simulink model "svpwm"  (R2020b)
settings: Solver=VariableStepAuto  StartTime=0.0  StopTime=10.0  RelTol=1e-3
libraries: simulink x1
settings Model: Creator=Administrator  LastModifiedBy=Administrator
settings DataIOCC: ReturnWorkspaceOutputs=off
settings DebuggingCC: ArithmeticOperatorsInVariantConditions=warning
settings SFSimCC: SimUseLocalCustomCode=off  CustomCodeUndefinedFunction=UseInterfaceOnly
settings RTWCC: RTWUseLocalCustomCode=off
settings CodeAppCC: StateflowObjectComments=on
settings SimscapeCC: SimscapeNormalizeSystem=off

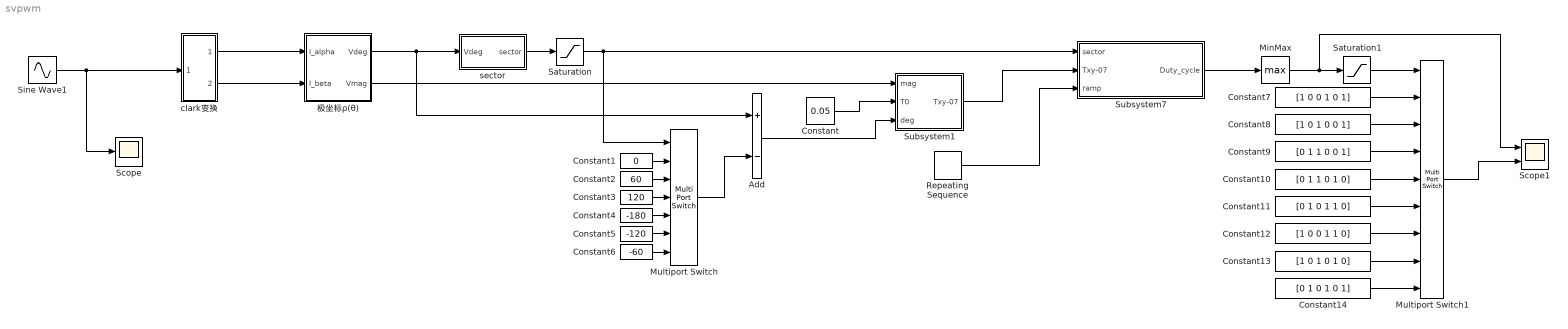
== system svpwm ==
  Add : Sum  Inputs=+-
  Constant : Constant  Value=0.05
  Constant1 : Constant  Value=0
  Constant10 : Constant  Value=[0 1 1 0 1 0]  VectorParams1D=off  SampleTime=-1
  Constant11 : Constant  Value=[0 1 0 1 1 0]  VectorParams1D=off  SampleTime=-1
  Constant12 : Constant  Value=[1 0 0 1 1 0]  VectorParams1D=off  SampleTime=-1
  Constant13 : Constant  Value=[1 0 1 0 1 0]  VectorParams1D=off  SampleTime=-1
  Constant14 : Constant  Value=[0 1 0 1 0 1]  VectorParams1D=off  SampleTime=-1
  Constant2 : Constant  Value=60
  Constant3 : Constant  Value=120
  Constant4 : Constant  Value=-180
  Constant5 : Constant  Value=-120
  Constant6 : Constant  Value=-60
  Constant7 : Constant  Value=[1 0 0 1 0 1]  VectorParams1D=off  SampleTime=-1
  Constant8 : Constant  Value=[1 0 1 0 0 1]  VectorParams1D=off  SampleTime=-1
  Constant9 : Constant  Value=[0 1 1 0 0 1]  VectorParams1D=off  SampleTime=-1
  MinMax : MinMax  Function=max
  Multiport Switch : MultiPortSwitch  Inputs=6
  Multiport Switch1 : MultiPortSwitch  Inputs=8
  Repeating Sequence : simulink/Sources/Repeating Sequence  rep_seq_t=[0 1e-4]  rep_seq_y=[0 1]
  Saturation : Saturate  UpperLimit=6  LowerLimit=1
  Saturation1 : Saturate  UpperLimit=8  LowerLimit=1
  Scope : Scope
  Scope1 : Scope  NumInputPorts=2
  Sine Wave1 : Sin  Amplitude=0.4  Frequency=2*pi*50  Phase=[0 -2*pi/3 2*pi/3]  SampleTime=1e-6
  Subsystem1 : Subsystem
  Subsystem7 : Subsystem
  clark变换 : Subsystem
  sector : Subsystem
  极坐标ρ(θ) : Subsystem
  wires:
  Sine Wave1/1 -> clark变换/1(I_abc), Scope/1
  clark变换/1(I_alpha) -> 极坐标ρ(θ)/1("I_alpha ")
  clark变换/2(I_beta) -> 极坐标ρ(θ)/2(I_beta)
  极坐标ρ(θ)/1(Vdeg) -> sector/1("Vdeg "), Add/1
  sector/1(sector) -> Saturation/1
  Saturation/1 -> Multiport Switch/1, Subsystem7/1(sector)
  Constant1/1 -> Multiport Switch/2
  Constant2/1 -> Multiport Switch/3
  Constant3/1 -> Multiport Switch/4
  Constant4/1 -> Multiport Switch/5
  Constant5/1 -> Multiport Switch/6
  Constant6/1 -> Multiport Switch/7
  Multiport Switch/1 -> Add/2
  极坐标ρ(θ)/2("Vmag ") -> Subsystem1/1(mag)
  Constant/1 -> Subsystem1/2("T0 ")
  Add/1 -> Subsystem1/3(deg)
  Subsystem1/1(Txy-07) -> Subsystem7/2(Txy-07)
  Repeating Sequence/1 -> Subsystem7/3(ramp)
  Subsystem7/1(Duty_cycle) -> MinMax/1
  MinMax/1 -> Scope1/1, Saturation1/1
  Saturation1/1 -> Multiport Switch1/1
  Constant7/1 -> Multiport Switch1/2
  Constant8/1 -> Multiport Switch1/3
  Constant14/1 -> Multiport Switch1/9
  Constant13/1 -> Multiport Switch1/8
  Constant12/1 -> Multiport Switch1/7
  Constant11/1 -> Multiport Switch1/6
  Constant10/1 -> Multiport Switch1/5
  Constant9/1 -> Multiport Switch1/4
  Multiport Switch1/1 -> Scope1/2

== system svpwm/Subsystem1 ==
  mag : Inport
  "T0 " : Inport  Port=2
  deg : Inport  Port=3
  Mux : Mux
  duty-cycles : Subsystem
  Txy-07 : Outport
  wires:
  duty-cycles/2(Ty) -> Mux/2
  duty-cycles/4(T7) -> Mux/4
  duty-cycles/1(Tx) -> Mux/1
  deg/1 -> duty-cycles/1(deg)
  "T0 "/1 -> duty-cycles/3("T0 ")
  Mux/1 -> Txy-07/1
  duty-cycles/3(T0) -> Mux/3
  mag/1 -> duty-cycles/2(mag)

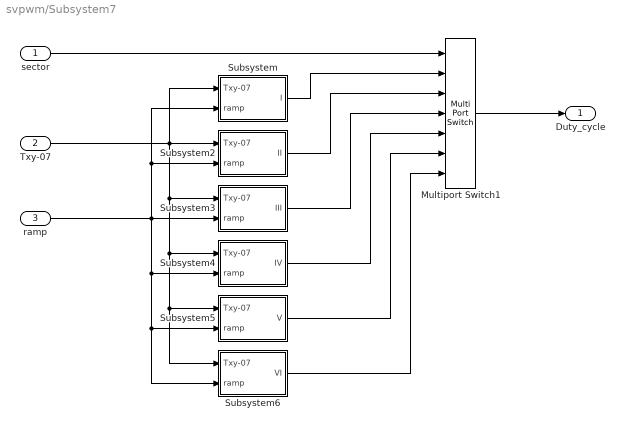
== system svpwm/Subsystem7 ==
  sector : Inport
  Txy-07 : Inport  Port=2
  ramp : Inport  Port=3
  Multiport Switch1 : MultiPortSwitch  Inputs=6
  Subsystem : Subsystem
  Subsystem2 : Subsystem
  Subsystem3 : Subsystem
  Subsystem4 : Subsystem
  Subsystem5 : Subsystem
  Subsystem6 : Subsystem
  Duty_cycle : Outport
  wires:
  Txy-07/1 -> Subsystem/1(Txy-07), Subsystem2/1(Txy-07), Subsystem3/1(Txy-07), Subsystem4/1(Txy-07), Subsystem5/1(Txy-07), Subsystem6/1(Txy-07)
  ramp/1 -> Subsystem/2(ramp), Subsystem2/2(ramp), Subsystem6/2(ramp), Subsystem5/2(ramp), Subsystem4/2(ramp), Subsystem3/2(ramp)
  Subsystem/1(I) -> Multiport Switch1/2
  Subsystem6/1(VI) -> Multiport Switch1/7
  Subsystem5/1(V) -> Multiport Switch1/6
  Subsystem3/1(III) -> Multiport Switch1/4
  Multiport Switch1/1 -> Duty_cycle/1
  Subsystem2/1(II) -> Multiport Switch1/3
  Subsystem4/1(IV) -> Multiport Switch1/5
  sector/1 -> Multiport Switch1/1

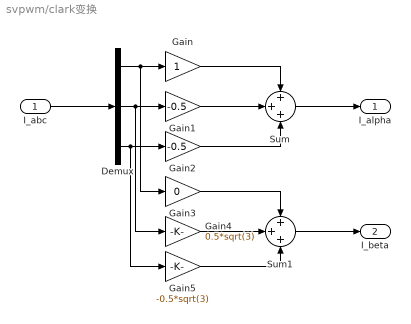
== system svpwm/clark变换 ==
  I_abc : Inport
  Demux : Demux  Outputs=3
  Gain : Gain
  Gain1 : Gain  Gain=-0.5
  Gain2 : Gain  Gain=-0.5
  Gain3 : Gain  Gain=0
  Gain4 : Gain  Gain=0.5*sqrt(3)
  Gain5 : Gain  Gain=-0.5*sqrt(3)
  Sum : Sum  Inputs=+++
  Sum1 : Sum  Inputs=+++
  I_alpha : Outport
  I_beta : Outport  Port=2
  wires:
  Gain5/1 -> Sum1/3
  Gain4/1 -> Sum1/2
  Gain1/1 -> Sum/2
  Gain2/1 -> Sum/3
  Demux/1 -> Gain/1, Gain3/1
  Sum/1 -> I_alpha/1
  I_abc/1 -> Demux/1
  Sum1/1 -> I_beta/1
  Demux/3 -> Gain5/1, Gain2/1
  Gain/1 -> Sum/1
  Demux/2 -> Gain4/1, Gain1/1
  Gain3/1 -> Sum1/1

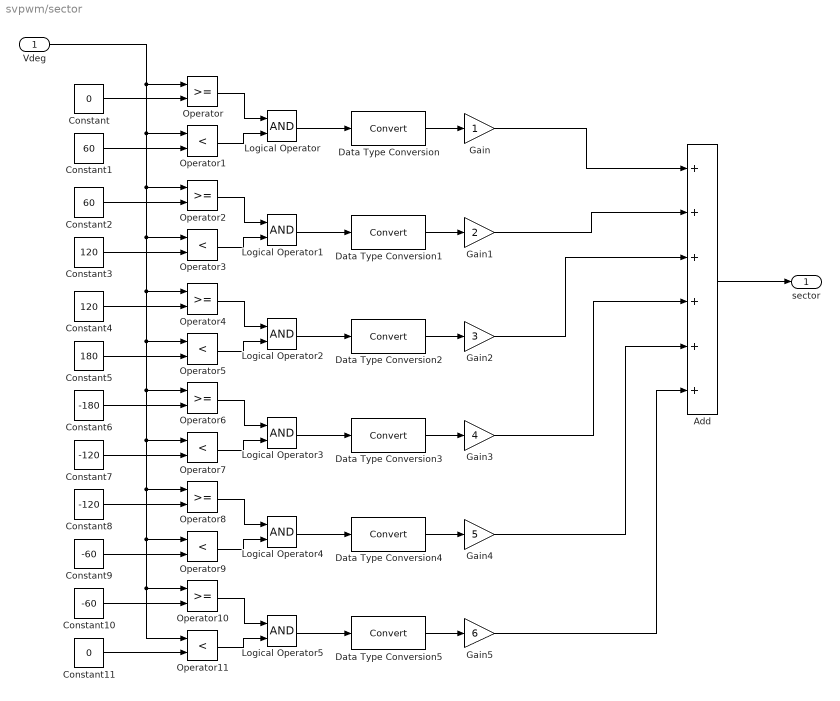
== system svpwm/sector ==
  "Vdeg " : Inport
  Add : Sum  Inputs=6
  Constant : Constant  Value=0
  Constant1 : Constant  Value=60
  Constant10 : Constant  Value=-60
  Constant11 : Constant  Value=0
  Constant2 : Constant  Value=60
  Constant3 : Constant  Value=120
  Constant4 : Constant  Value=120
  Constant5 : Constant  Value=180
  Constant6 : Constant  Value=-180
  Constant7 : Constant  Value=-120
  Constant8 : Constant  Value=-120
  Constant9 : Constant  Value=-60
  Data Type Conversion{,1..5} (6 alike) : DataTypeConversion
  Gain : Gain
  Gain1 : Gain  Gain=2
  Gain2 : Gain  Gain=3
  Gain3 : Gain  Gain=4
  Gain4 : Gain  Gain=5
  Gain5 : Gain  Gain=6
  Logical Operator{,1..5} (6 alike) : Logic  AllPortsSameDT=off  OutDataTypeStr=boolean
  Operator{,2,4,6,8,10} (6 alike) : RelationalOperator  OutDataTypeStr=boolean  RndMeth=Simplest
  Operator{1,3,5,7,9,11} (6 alike) : RelationalOperator  Operator=<  OutDataTypeStr=boolean  RndMeth=Simplest
  sector : Outport
  wires:
  Gain3/1 -> Add/4
  Gain1/1 -> Add/2
  Operator10/1 -> Logical Operator5/1
  Operator11/1 -> Logical Operator5/2
  "Vdeg "/1 -> Operator2/1, Operator6/1, Operator10/1, Operator11/1, Operator9/1, Operator8/1, Operator7/1, Operator5/1, Operator4/1, Operator3/1, Operator1/1, Operator/1
  Constant10/1 -> Operator10/2
  Logical Operator5/1 -> Data Type Conversion5/1
  Data Type Conversion5/1 -> Gain5/1
  Constant2/1 -> Operator2/2
  Operator2/1 -> Logical Operator1/1
  Constant3/1 -> Operator3/2
  Logical Operator1/1 -> Data Type Conversion1/1
  Operator3/1 -> Logical Operator1/2
  Data Type Conversion1/1 -> Gain1/1
  Logical Operator/1 -> Data Type Conversion/1
  Constant11/1 -> Operator11/2
  Constant/1 -> Operator/2
  Operator/1 -> Logical Operator/1
  Constant1/1 -> Operator1/2
  Gain/1 -> Add/1
  Operator1/1 -> Logical Operator/2
  Operator4/1 -> Logical Operator2/1
  Logical Operator2/1 -> Data Type Conversion2/1
  Constant5/1 -> Operator5/2
  Constant4/1 -> Operator4/2
  Operator5/1 -> Logical Operator2/2
  Data Type Conversion2/1 -> Gain2/1
  Constant7/1 -> Operator7/2
  Operator6/1 -> Logical Operator3/1
  Data Type Conversion3/1 -> Gain3/1
  Constant6/1 -> Operator6/2
  Operator7/1 -> Logical Operator3/2
  Logical Operator3/1 -> Data Type Conversion3/1
  Gain4/1 -> Add/5
  Gain5/1 -> Add/6
  Gain2/1 -> Add/3
  Data Type Conversion/1 -> Gain/1
  Add/1 -> sector/1
  Constant9/1 -> Operator9/2
  Operator8/1 -> Logical Operator4/1
  Operator9/1 -> Logical Operator4/2
  Data Type Conversion4/1 -> Gain4/1
  Logical Operator4/1 -> Data Type Conversion4/1
  Constant8/1 -> Operator8/2

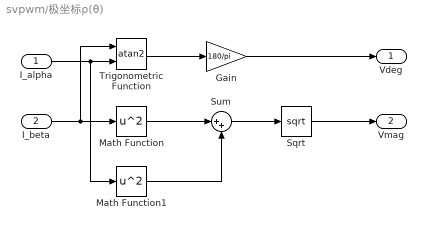
== system svpwm/极坐标ρ(θ) ==
  "I_alpha " : Inport
  I_beta : Inport  Port=2
  Gain : Gain  Gain=180/pi
  Math Function : Math  Operator=square  SignedPower=on  SaturateOnIntegerOverflow=on
  Math Function1 : Math  Operator=square  SignedPower=on  SaturateOnIntegerOverflow=on
  Sqrt : Sqrt  SaturateOnIntegerOverflow=on
  Sum : Sum  Inputs=|++
  Trigonometric Function : Trigonometry  Operator=atan2
  Vdeg : Outport
  "Vmag " : Outport  Port=2
  wires:
  "I_alpha "/1 -> Math Function1/1, Trigonometric Function/2
  I_beta/1 -> Trigonometric Function/1, Math Function/1
  Math Function/1 -> Sum/1
  Math Function1/1 -> Sum/2
  Sum/1 -> Sqrt/1
  Gain/1 -> Vdeg/1
  Trigonometric Function/1 -> Gain/1
  Sqrt/1 -> "Vmag "/1

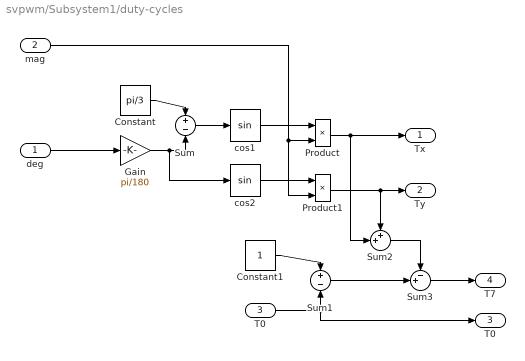
== system svpwm/Subsystem1/duty-cycles ==
  deg : Inport
  mag : Inport  Port=2
  "T0 " : Inport  Port=3
  Constant : Constant  Value=pi/3
  Constant1 : Constant
  Gain : Gain  Gain=pi/180
  Product : Product
  Product1 : Product
  Sum : Sum  Inputs=+|-
  Sum1 : Sum  Inputs=+-
  Sum2 : Sum  Inputs=++|
  Sum3 : Sum  Inputs=-+|
  cos1 : Trigonometry
  cos2 : Trigonometry
  Tx : Outport
  Ty : Outport  Port=2
  T0 : Outport  Port=3
  T7 : Outport  Port=4
  wires:
  Gain/1 -> cos2/1, Sum/2
  cos1/1 -> Product/1
  Sum/1 -> cos1/1
  mag/1 -> Product1/2, Product/2
  deg/1 -> Gain/1
  Product1/1 -> Sum2/1, Ty/1
  Product/1 -> Sum2/2, Tx/1
  cos2/1 -> Product1/1
  Constant/1 -> Sum/1
  Constant1/1 -> Sum1/1
  "T0 "/1 -> Sum1/2, T0/1
  Sum1/1 -> Sum3/2
  Sum2/1 -> Sum3/1
  Sum3/1 -> T7/1

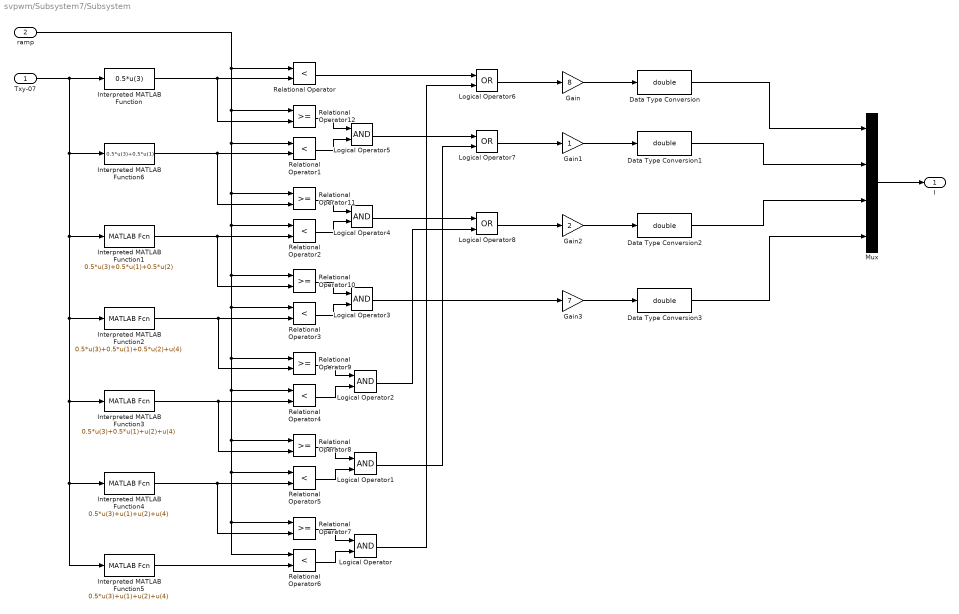
== system svpwm/Subsystem7/Subsystem ==
  Txy-07 : Inport
  ramp : Inport  Port=2
  Data Type Conversion{,1..3} (4 alike) : DataTypeConversion  OutDataTypeStr=double
  Gain : Gain  Gain=8
  Gain1 : Gain
  Gain2 : Gain  Gain=2
  Gain3 : Gain  Gain=7
  Interpreted MATLAB Function : MATLABFcn  MATLABFcn=0.5*u(3)
  Interpreted MATLAB Function1 : MATLABFcn  MATLABFcn=0.5*u(3)+0.5*u(1)+0.5*u(2)
  Interpreted MATLAB Function2 : MATLABFcn  MATLABFcn=0.5*u(3)+0.5*u(1)+0.5*u(2)+u(4)
  Interpreted MATLAB Function3 : MATLABFcn  MATLABFcn=0.5*u(3)+0.5*u(1)+u(2)+u(4)
  Interpreted MATLAB Function4 : MATLABFcn  MATLABFcn=0.5*u(3)+u(1)+u(2)+u(4)
  Interpreted MATLAB Function5 : MATLABFcn  MATLABFcn=0.5*u(3)+u(1)+u(2)+u(4)
  Interpreted MATLAB Function6 : MATLABFcn  MATLABFcn=0.5*u(3)+0.5*u(1)
  Logical Operator{,1..5} (6 alike) : Logic  AllPortsSameDT=off  OutDataTypeStr=boolean
  Logical Operator6 : Logic  Operator=OR  AllPortsSameDT=off  OutDataTypeStr=boolean
  Logical Operator7 : Logic  Operator=OR  AllPortsSameDT=off  OutDataTypeStr=boolean
  Logical Operator8 : Logic  Operator=OR  AllPortsSameDT=off  OutDataTypeStr=boolean
  Mux : Mux
  Relational Operator{,1..6} (7 alike) : RelationalOperator  Operator=<  OutDataTypeStr=boolean  RndMeth=Simplest
  Relational Operator{7..12} (6 alike) : RelationalOperator  OutDataTypeStr=boolean  RndMeth=Simplest
  I : Outport
  wires:
  Txy-07/1 -> Interpreted MATLAB Function5/1, Interpreted MATLAB Function4/1, Interpreted MATLAB Function3/1, Interpreted MATLAB Function2/1, Interpreted MATLAB Function1/1, Interpreted MATLAB Function6/1, Interpreted MATLAB Function/1
  Interpreted MATLAB Function/1 -> Relational Operator12/2, Relational Operator/2
  Interpreted MATLAB Function6/1 -> Relational Operator11/2, Relational Operator1/2
  Interpreted MATLAB Function1/1 -> Relational Operator10/2, Relational Operator2/2
  Interpreted MATLAB Function2/1 -> Relational Operator9/2, Relational Operator3/2
  Interpreted MATLAB Function3/1 -> Relational Operator8/2, Relational Operator4/2
  Interpreted MATLAB Function5/1 -> Relational Operator6/2
  Interpreted MATLAB Function4/1 -> Relational Operator7/2, Relational Operator5/2
  Relational Operator7/1 -> Logical Operator/1
  Relational Operator6/1 -> Logical Operator/2
  Relational Operator12/1 -> Logical Operator5/1
  Relational Operator1/1 -> Logical Operator5/2
  Relational Operator11/1 -> Logical Operator4/1
  Relational Operator2/1 -> Logical Operator4/2
  Relational Operator10/1 -> Logical Operator3/1
  Relational Operator3/1 -> Logical Operator3/2
  Relational Operator9/1 -> Logical Operator2/1
  Relational Operator4/1 -> Logical Operator2/2
  Relational Operator8/1 -> Logical Operator1/1
  Relational Operator5/1 -> Logical Operator1/2
  ramp/1 -> Relational Operator12/1, Relational Operator11/1, Relational Operator10/1, Relational Operator9/1, Relational Operator8/1, Relational Operator7/1, Relational Operator6/1, Relational Operator5/1, Relational Operator4/1, Relational Operator3/1, Relational Operator2/1, Relational Operator1/1, Relational Operator/1
  Relational Operator/1 -> Logical Operator6/1
  Logical Operator/1 -> Logical Operator6/2
  Logical Operator5/1 -> Logical Operator7/1
  Logical Operator1/1 -> Logical Operator7/2
  Logical Operator4/1 -> Logical Operator8/1
  Logical Operator2/1 -> Logical Operator8/2
  Logical Operator6/1 -> Gain/1
  Logical Operator7/1 -> Gain1/1
  Logical Operator8/1 -> Gain2/1
  Logical Operator3/1 -> Gain3/1
  Gain3/1 -> Data Type Conversion3/1
  Gain2/1 -> Data Type Conversion2/1
  Gain1/1 -> Data Type Conversion1/1
  Gain/1 -> Data Type Conversion/1
  Data Type Conversion/1 -> Mux/1
  Data Type Conversion1/1 -> Mux/2
  Data Type Conversion2/1 -> Mux/3
  Data Type Conversion3/1 -> Mux/4
  Mux/1 -> I/1

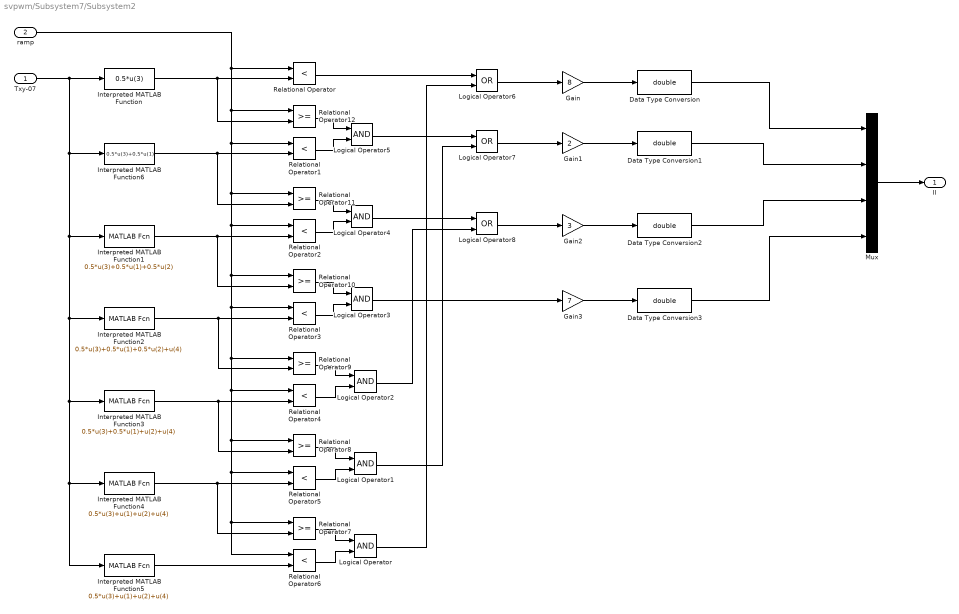
== system svpwm/Subsystem7/Subsystem2 ==
  Txy-07 : Inport
  ramp : Inport  Port=2
  Data Type Conversion{,1..3} (4 alike) : DataTypeConversion  OutDataTypeStr=double
  Gain : Gain  Gain=8
  Gain1 : Gain  Gain=2
  Gain2 : Gain  Gain=3
  Gain3 : Gain  Gain=7
  Interpreted MATLAB Function : MATLABFcn  MATLABFcn=0.5*u(3)
  Interpreted MATLAB Function1 : MATLABFcn  MATLABFcn=0.5*u(3)+0.5*u(1)+0.5*u(2)
  Interpreted MATLAB Function2 : MATLABFcn  MATLABFcn=0.5*u(3)+0.5*u(1)+0.5*u(2)+u(4)
  Interpreted MATLAB Function3 : MATLABFcn  MATLABFcn=0.5*u(3)+0.5*u(1)+u(2)+u(4)
  Interpreted MATLAB Function4 : MATLABFcn  MATLABFcn=0.5*u(3)+u(1)+u(2)+u(4)
  Interpreted MATLAB Function5 : MATLABFcn  MATLABFcn=0.5*u(3)+u(1)+u(2)+u(4)
  Interpreted MATLAB Function6 : MATLABFcn  MATLABFcn=0.5*u(3)+0.5*u(1)
  Logical Operator{,1..5} (6 alike) : Logic  AllPortsSameDT=off  OutDataTypeStr=boolean
  Logical Operator6 : Logic  Operator=OR  AllPortsSameDT=off  OutDataTypeStr=boolean
  Logical Operator7 : Logic  Operator=OR  AllPortsSameDT=off  OutDataTypeStr=boolean
  Logical Operator8 : Logic  Operator=OR  AllPortsSameDT=off  OutDataTypeStr=boolean
  Mux : Mux
  Relational Operator{,1..6} (7 alike) : RelationalOperator  Operator=<  OutDataTypeStr=boolean  RndMeth=Simplest
  Relational Operator{7..12} (6 alike) : RelationalOperator  OutDataTypeStr=boolean  RndMeth=Simplest
  II : Outport
  wires:
  Mux/1 -> II/1
  Data Type Conversion3/1 -> Mux/4
  Data Type Conversion2/1 -> Mux/3
  Data Type Conversion1/1 -> Mux/2
  Data Type Conversion/1 -> Mux/1
  Gain/1 -> Data Type Conversion/1
  Gain1/1 -> Data Type Conversion1/1
  Gain2/1 -> Data Type Conversion2/1
  Gain3/1 -> Data Type Conversion3/1
  Logical Operator3/1 -> Gain3/1
  Logical Operator8/1 -> Gain2/1
  Logical Operator7/1 -> Gain1/1
  Logical Operator6/1 -> Gain/1
  Logical Operator2/1 -> Logical Operator8/2
  Logical Operator4/1 -> Logical Operator8/1
  Logical Operator1/1 -> Logical Operator7/2
  Logical Operator5/1 -> Logical Operator7/1
  Logical Operator/1 -> Logical Operator6/2
  Relational Operator/1 -> Logical Operator6/1
  ramp/1 -> Relational Operator/1, Relational Operator1/1, Relational Operator2/1, Relational Operator3/1, Relational Operator4/1, Relational Operator5/1, Relational Operator6/1, Relational Operator7/1, Relational Operator8/1, Relational Operator9/1, Relational Operator10/1, Relational Operator11/1, Relational Operator12/1
  Relational Operator5/1 -> Logical Operator1/2
  Relational Operator8/1 -> Logical Operator1/1
  Relational Operator4/1 -> Logical Operator2/2
  Relational Operator9/1 -> Logical Operator2/1
  Relational Operator3/1 -> Logical Operator3/2
  Relational Operator10/1 -> Logical Operator3/1
  Relational Operator2/1 -> Logical Operator4/2
  Relational Operator11/1 -> Logical Operator4/1
  Relational Operator1/1 -> Logical Operator5/2
  Relational Operator12/1 -> Logical Operator5/1
  Relational Operator6/1 -> Logical Operator/2
  Relational Operator7/1 -> Logical Operator/1
  Interpreted MATLAB Function4/1 -> Relational Operator5/2, Relational Operator7/2
  Interpreted MATLAB Function5/1 -> Relational Operator6/2
  Interpreted MATLAB Function3/1 -> Relational Operator4/2, Relational Operator8/2
  Interpreted MATLAB Function2/1 -> Relational Operator3/2, Relational Operator9/2
  Interpreted MATLAB Function1/1 -> Relational Operator2/2, Relational Operator10/2
  Interpreted MATLAB Function6/1 -> Relational Operator1/2, Relational Operator11/2
  Interpreted MATLAB Function/1 -> Relational Operator/2, Relational Operator12/2
  Txy-07/1 -> Interpreted MATLAB Function/1, Interpreted MATLAB Function6/1, Interpreted MATLAB Function1/1, Interpreted MATLAB Function2/1, Interpreted MATLAB Function3/1, Interpreted MATLAB Function4/1, Interpreted MATLAB Function5/1

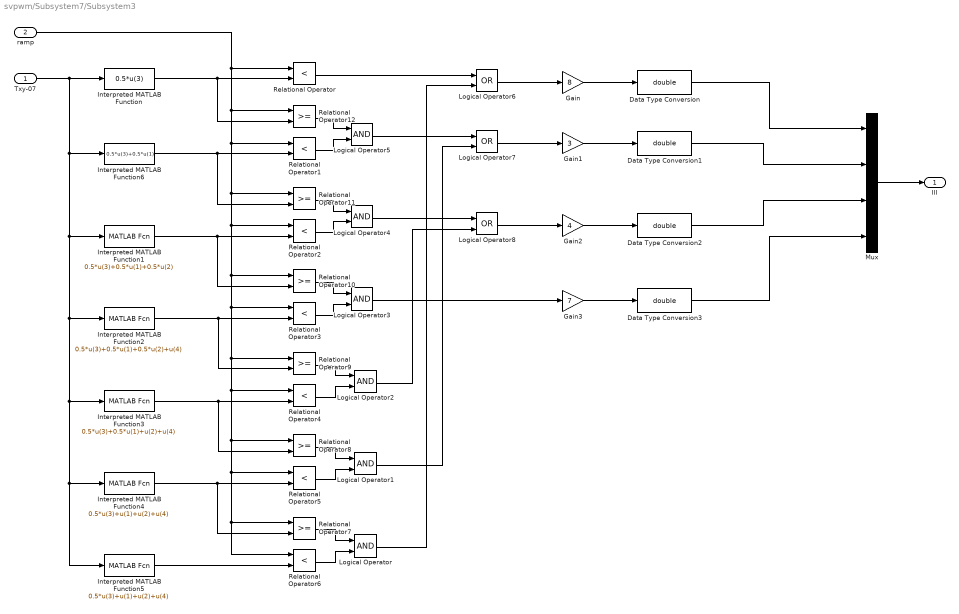
== system svpwm/Subsystem7/Subsystem3 ==
  Txy-07 : Inport
  ramp : Inport  Port=2
  Data Type Conversion{,1..3} (4 alike) : DataTypeConversion  OutDataTypeStr=double
  Gain : Gain  Gain=8
  Gain1 : Gain  Gain=3
  Gain2 : Gain  Gain=4
  Gain3 : Gain  Gain=7
  Interpreted MATLAB Function : MATLABFcn  MATLABFcn=0.5*u(3)
  Interpreted MATLAB Function1 : MATLABFcn  MATLABFcn=0.5*u(3)+0.5*u(1)+0.5*u(2)
  Interpreted MATLAB Function2 : MATLABFcn  MATLABFcn=0.5*u(3)+0.5*u(1)+0.5*u(2)+u(4)
  Interpreted MATLAB Function3 : MATLABFcn  MATLABFcn=0.5*u(3)+0.5*u(1)+u(2)+u(4)
  Interpreted MATLAB Function4 : MATLABFcn  MATLABFcn=0.5*u(3)+u(1)+u(2)+u(4)
  Interpreted MATLAB Function5 : MATLABFcn  MATLABFcn=0.5*u(3)+u(1)+u(2)+u(4)
  Interpreted MATLAB Function6 : MATLABFcn  MATLABFcn=0.5*u(3)+0.5*u(1)
  Logical Operator{,1..5} (6 alike) : Logic  AllPortsSameDT=off  OutDataTypeStr=boolean
  Logical Operator6 : Logic  Operator=OR  AllPortsSameDT=off  OutDataTypeStr=boolean
  Logical Operator7 : Logic  Operator=OR  AllPortsSameDT=off  OutDataTypeStr=boolean
  Logical Operator8 : Logic  Operator=OR  AllPortsSameDT=off  OutDataTypeStr=boolean
  Mux : Mux
  Relational Operator{,1..6} (7 alike) : RelationalOperator  Operator=<  OutDataTypeStr=boolean  RndMeth=Simplest
  Relational Operator{7..12} (6 alike) : RelationalOperator  OutDataTypeStr=boolean  RndMeth=Simplest
  III : Outport
  wires:
  Txy-07/1 -> Interpreted MATLAB Function5/1, Interpreted MATLAB Function4/1, Interpreted MATLAB Function3/1, Interpreted MATLAB Function2/1, Interpreted MATLAB Function1/1, Interpreted MATLAB Function6/1, Interpreted MATLAB Function/1
  Interpreted MATLAB Function/1 -> Relational Operator12/2, Relational Operator/2
  Interpreted MATLAB Function6/1 -> Relational Operator11/2, Relational Operator1/2
  Interpreted MATLAB Function1/1 -> Relational Operator10/2, Relational Operator2/2
  Interpreted MATLAB Function2/1 -> Relational Operator9/2, Relational Operator3/2
  Interpreted MATLAB Function3/1 -> Relational Operator8/2, Relational Operator4/2
  Interpreted MATLAB Function5/1 -> Relational Operator6/2
  Interpreted MATLAB Function4/1 -> Relational Operator7/2, Relational Operator5/2
  Relational Operator7/1 -> Logical Operator/1
  Relational Operator6/1 -> Logical Operator/2
  Relational Operator12/1 -> Logical Operator5/1
  Relational Operator1/1 -> Logical Operator5/2
  Relational Operator11/1 -> Logical Operator4/1
  Relational Operator2/1 -> Logical Operator4/2
  Relational Operator10/1 -> Logical Operator3/1
  Relational Operator3/1 -> Logical Operator3/2
  Relational Operator9/1 -> Logical Operator2/1
  Relational Operator4/1 -> Logical Operator2/2
  Relational Operator8/1 -> Logical Operator1/1
  Relational Operator5/1 -> Logical Operator1/2
  ramp/1 -> Relational Operator12/1, Relational Operator11/1, Relational Operator10/1, Relational Operator9/1, Relational Operator8/1, Relational Operator7/1, Relational Operator6/1, Relational Operator5/1, Relational Operator4/1, Relational Operator3/1, Relational Operator2/1, Relational Operator1/1, Relational Operator/1
  Relational Operator/1 -> Logical Operator6/1
  Logical Operator/1 -> Logical Operator6/2
  Logical Operator5/1 -> Logical Operator7/1
  Logical Operator1/1 -> Logical Operator7/2
  Logical Operator4/1 -> Logical Operator8/1
  Logical Operator2/1 -> Logical Operator8/2
  Logical Operator6/1 -> Gain/1
  Logical Operator7/1 -> Gain1/1
  Logical Operator8/1 -> Gain2/1
  Logical Operator3/1 -> Gain3/1
  Gain3/1 -> Data Type Conversion3/1
  Gain2/1 -> Data Type Conversion2/1
  Gain1/1 -> Data Type Conversion1/1
  Gain/1 -> Data Type Conversion/1
  Data Type Conversion/1 -> Mux/1
  Data Type Conversion1/1 -> Mux/2
  Data Type Conversion2/1 -> Mux/3
  Data Type Conversion3/1 -> Mux/4
  Mux/1 -> III/1

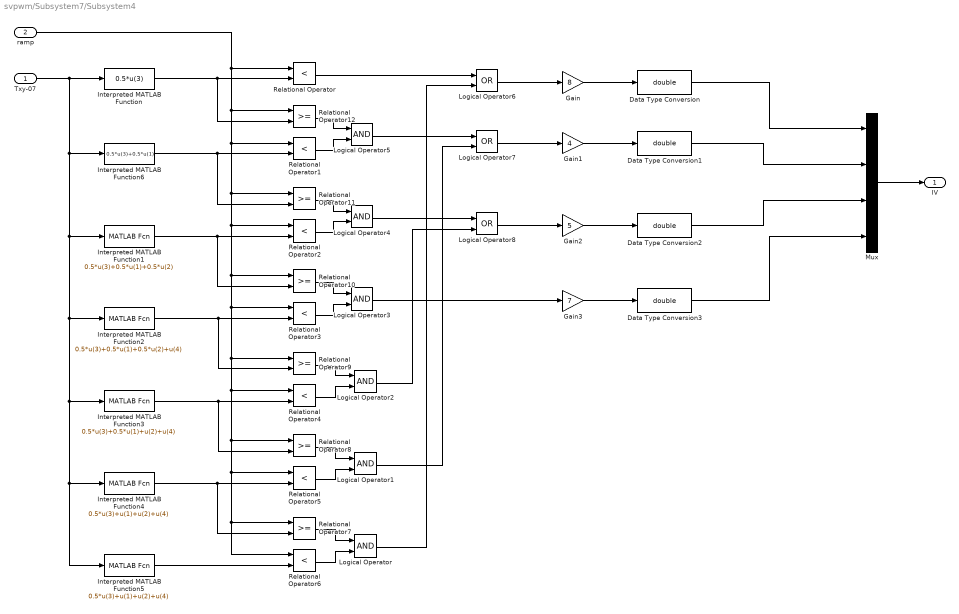
== system svpwm/Subsystem7/Subsystem4 ==
  Txy-07 : Inport
  ramp : Inport  Port=2
  Data Type Conversion{,1..3} (4 alike) : DataTypeConversion  OutDataTypeStr=double
  Gain : Gain  Gain=8
  Gain1 : Gain  Gain=4
  Gain2 : Gain  Gain=5
  Gain3 : Gain  Gain=7
  Interpreted MATLAB Function : MATLABFcn  MATLABFcn=0.5*u(3)
  Interpreted MATLAB Function1 : MATLABFcn  MATLABFcn=0.5*u(3)+0.5*u(1)+0.5*u(2)
  Interpreted MATLAB Function2 : MATLABFcn  MATLABFcn=0.5*u(3)+0.5*u(1)+0.5*u(2)+u(4)
  Interpreted MATLAB Function3 : MATLABFcn  MATLABFcn=0.5*u(3)+0.5*u(1)+u(2)+u(4)
  Interpreted MATLAB Function4 : MATLABFcn  MATLABFcn=0.5*u(3)+u(1)+u(2)+u(4)
  Interpreted MATLAB Function5 : MATLABFcn  MATLABFcn=0.5*u(3)+u(1)+u(2)+u(4)
  Interpreted MATLAB Function6 : MATLABFcn  MATLABFcn=0.5*u(3)+0.5*u(1)
  Logical Operator{,1..5} (6 alike) : Logic  AllPortsSameDT=off  OutDataTypeStr=boolean
  Logical Operator6 : Logic  Operator=OR  AllPortsSameDT=off  OutDataTypeStr=boolean
  Logical Operator7 : Logic  Operator=OR  AllPortsSameDT=off  OutDataTypeStr=boolean
  Logical Operator8 : Logic  Operator=OR  AllPortsSameDT=off  OutDataTypeStr=boolean
  Mux : Mux
  Relational Operator{,1..6} (7 alike) : RelationalOperator  Operator=<  OutDataTypeStr=boolean  RndMeth=Simplest
  Relational Operator{7..12} (6 alike) : RelationalOperator  OutDataTypeStr=boolean  RndMeth=Simplest
  IV : Outport
  wires:
  Mux/1 -> IV/1
  Data Type Conversion3/1 -> Mux/4
  Data Type Conversion2/1 -> Mux/3
  Data Type Conversion1/1 -> Mux/2
  Data Type Conversion/1 -> Mux/1
  Gain/1 -> Data Type Conversion/1
  Gain1/1 -> Data Type Conversion1/1
  Gain2/1 -> Data Type Conversion2/1
  Gain3/1 -> Data Type Conversion3/1
  Logical Operator3/1 -> Gain3/1
  Logical Operator8/1 -> Gain2/1
  Logical Operator7/1 -> Gain1/1
  Logical Operator6/1 -> Gain/1
  Logical Operator2/1 -> Logical Operator8/2
  Logical Operator4/1 -> Logical Operator8/1
  Logical Operator1/1 -> Logical Operator7/2
  Logical Operator5/1 -> Logical Operator7/1
  Logical Operator/1 -> Logical Operator6/2
  Relational Operator/1 -> Logical Operator6/1
  ramp/1 -> Relational Operator/1, Relational Operator1/1, Relational Operator2/1, Relational Operator3/1, Relational Operator4/1, Relational Operator5/1, Relational Operator6/1, Relational Operator7/1, Relational Operator8/1, Relational Operator9/1, Relational Operator10/1, Relational Operator11/1, Relational Operator12/1
  Relational Operator5/1 -> Logical Operator1/2
  Relational Operator8/1 -> Logical Operator1/1
  Relational Operator4/1 -> Logical Operator2/2
  Relational Operator9/1 -> Logical Operator2/1
  Relational Operator3/1 -> Logical Operator3/2
  Relational Operator10/1 -> Logical Operator3/1
  Relational Operator2/1 -> Logical Operator4/2
  Relational Operator11/1 -> Logical Operator4/1
  Relational Operator1/1 -> Logical Operator5/2
  Relational Operator12/1 -> Logical Operator5/1
  Relational Operator6/1 -> Logical Operator/2
  Relational Operator7/1 -> Logical Operator/1
  Interpreted MATLAB Function4/1 -> Relational Operator5/2, Relational Operator7/2
  Interpreted MATLAB Function5/1 -> Relational Operator6/2
  Interpreted MATLAB Function3/1 -> Relational Operator4/2, Relational Operator8/2
  Interpreted MATLAB Function2/1 -> Relational Operator3/2, Relational Operator9/2
  Interpreted MATLAB Function1/1 -> Relational Operator2/2, Relational Operator10/2
  Interpreted MATLAB Function6/1 -> Relational Operator1/2, Relational Operator11/2
  Interpreted MATLAB Function/1 -> Relational Operator/2, Relational Operator12/2
  Txy-07/1 -> Interpreted MATLAB Function/1, Interpreted MATLAB Function6/1, Interpreted MATLAB Function1/1, Interpreted MATLAB Function2/1, Interpreted MATLAB Function3/1, Interpreted MATLAB Function4/1, Interpreted MATLAB Function5/1

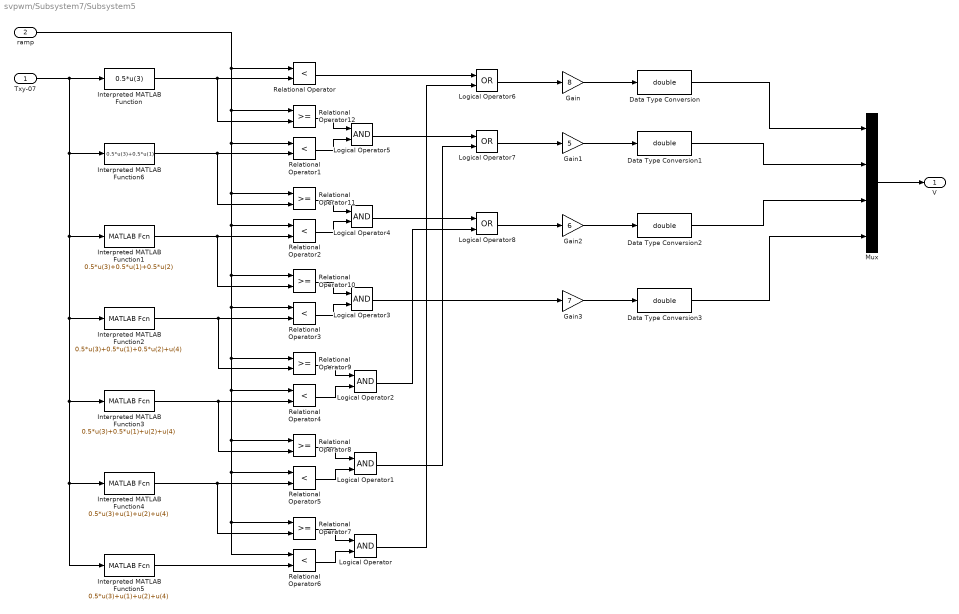
== system svpwm/Subsystem7/Subsystem5 ==
  Txy-07 : Inport
  ramp : Inport  Port=2
  Data Type Conversion{,1..3} (4 alike) : DataTypeConversion  OutDataTypeStr=double
  Gain : Gain  Gain=8
  Gain1 : Gain  Gain=5
  Gain2 : Gain  Gain=6
  Gain3 : Gain  Gain=7
  Interpreted MATLAB Function : MATLABFcn  MATLABFcn=0.5*u(3)
  Interpreted MATLAB Function1 : MATLABFcn  MATLABFcn=0.5*u(3)+0.5*u(1)+0.5*u(2)
  Interpreted MATLAB Function2 : MATLABFcn  MATLABFcn=0.5*u(3)+0.5*u(1)+0.5*u(2)+u(4)
  Interpreted MATLAB Function3 : MATLABFcn  MATLABFcn=0.5*u(3)+0.5*u(1)+u(2)+u(4)
  Interpreted MATLAB Function4 : MATLABFcn  MATLABFcn=0.5*u(3)+u(1)+u(2)+u(4)
  Interpreted MATLAB Function5 : MATLABFcn  MATLABFcn=0.5*u(3)+u(1)+u(2)+u(4)
  Interpreted MATLAB Function6 : MATLABFcn  MATLABFcn=0.5*u(3)+0.5*u(1)
  Logical Operator{,1..5} (6 alike) : Logic  AllPortsSameDT=off  OutDataTypeStr=boolean
  Logical Operator6 : Logic  Operator=OR  AllPortsSameDT=off  OutDataTypeStr=boolean
  Logical Operator7 : Logic  Operator=OR  AllPortsSameDT=off  OutDataTypeStr=boolean
  Logical Operator8 : Logic  Operator=OR  AllPortsSameDT=off  OutDataTypeStr=boolean
  Mux : Mux
  Relational Operator{,1..6} (7 alike) : RelationalOperator  Operator=<  OutDataTypeStr=boolean  RndMeth=Simplest
  Relational Operator{7..12} (6 alike) : RelationalOperator  OutDataTypeStr=boolean  RndMeth=Simplest
  V : Outport
  wires:
  Txy-07/1 -> Interpreted MATLAB Function5/1, Interpreted MATLAB Function4/1, Interpreted MATLAB Function3/1, Interpreted MATLAB Function2/1, Interpreted MATLAB Function1/1, Interpreted MATLAB Function6/1, Interpreted MATLAB Function/1
  Interpreted MATLAB Function/1 -> Relational Operator12/2, Relational Operator/2
  Interpreted MATLAB Function6/1 -> Relational Operator11/2, Relational Operator1/2
  Interpreted MATLAB Function1/1 -> Relational Operator10/2, Relational Operator2/2
  Interpreted MATLAB Function2/1 -> Relational Operator9/2, Relational Operator3/2
  Interpreted MATLAB Function3/1 -> Relational Operator8/2, Relational Operator4/2
  Interpreted MATLAB Function5/1 -> Relational Operator6/2
  Interpreted MATLAB Function4/1 -> Relational Operator7/2, Relational Operator5/2
  Relational Operator7/1 -> Logical Operator/1
  Relational Operator6/1 -> Logical Operator/2
  Relational Operator12/1 -> Logical Operator5/1
  Relational Operator1/1 -> Logical Operator5/2
  Relational Operator11/1 -> Logical Operator4/1
  Relational Operator2/1 -> Logical Operator4/2
  Relational Operator10/1 -> Logical Operator3/1
  Relational Operator3/1 -> Logical Operator3/2
  Relational Operator9/1 -> Logical Operator2/1
  Relational Operator4/1 -> Logical Operator2/2
  Relational Operator8/1 -> Logical Operator1/1
  Relational Operator5/1 -> Logical Operator1/2
  ramp/1 -> Relational Operator12/1, Relational Operator11/1, Relational Operator10/1, Relational Operator9/1, Relational Operator8/1, Relational Operator7/1, Relational Operator6/1, Relational Operator5/1, Relational Operator4/1, Relational Operator3/1, Relational Operator2/1, Relational Operator1/1, Relational Operator/1
  Relational Operator/1 -> Logical Operator6/1
  Logical Operator/1 -> Logical Operator6/2
  Logical Operator5/1 -> Logical Operator7/1
  Logical Operator1/1 -> Logical Operator7/2
  Logical Operator4/1 -> Logical Operator8/1
  Logical Operator2/1 -> Logical Operator8/2
  Logical Operator6/1 -> Gain/1
  Logical Operator7/1 -> Gain1/1
  Logical Operator8/1 -> Gain2/1
  Logical Operator3/1 -> Gain3/1
  Gain3/1 -> Data Type Conversion3/1
  Gain2/1 -> Data Type Conversion2/1
  Gain1/1 -> Data Type Conversion1/1
  Gain/1 -> Data Type Conversion/1
  Data Type Conversion/1 -> Mux/1
  Data Type Conversion1/1 -> Mux/2
  Data Type Conversion2/1 -> Mux/3
  Data Type Conversion3/1 -> Mux/4
  Mux/1 -> V/1

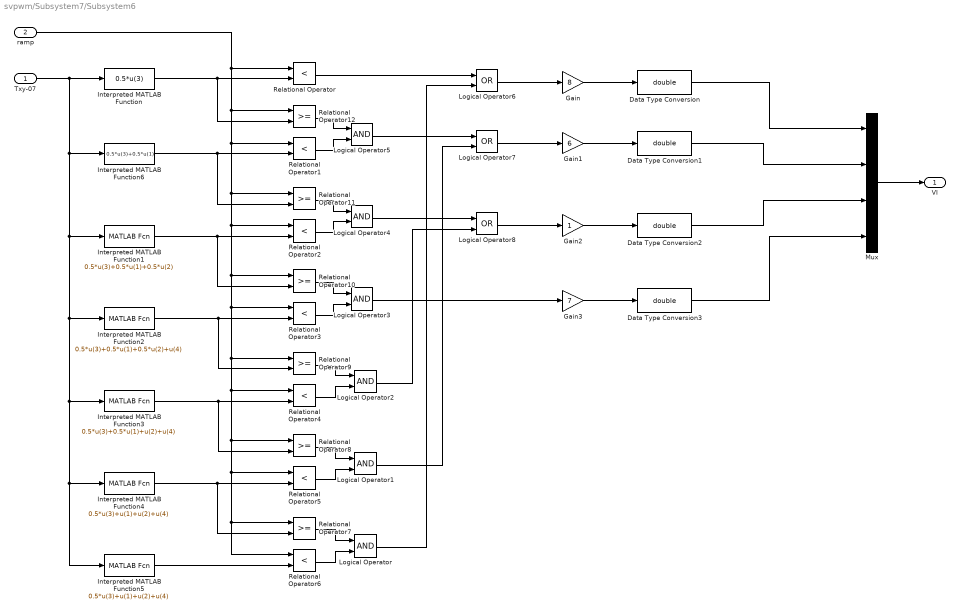
== system svpwm/Subsystem7/Subsystem6 ==
  Txy-07 : Inport
  ramp : Inport  Port=2
  Data Type Conversion{,1..3} (4 alike) : DataTypeConversion  OutDataTypeStr=double
  Gain : Gain  Gain=8
  Gain1 : Gain  Gain=6
  Gain2 : Gain
  Gain3 : Gain  Gain=7
  Interpreted MATLAB Function : MATLABFcn  MATLABFcn=0.5*u(3)
  Interpreted MATLAB Function1 : MATLABFcn  MATLABFcn=0.5*u(3)+0.5*u(1)+0.5*u(2)
  Interpreted MATLAB Function2 : MATLABFcn  MATLABFcn=0.5*u(3)+0.5*u(1)+0.5*u(2)+u(4)
  Interpreted MATLAB Function3 : MATLABFcn  MATLABFcn=0.5*u(3)+0.5*u(1)+u(2)+u(4)
  Interpreted MATLAB Function4 : MATLABFcn  MATLABFcn=0.5*u(3)+u(1)+u(2)+u(4)
  Interpreted MATLAB Function5 : MATLABFcn  MATLABFcn=0.5*u(3)+u(1)+u(2)+u(4)
  Interpreted MATLAB Function6 : MATLABFcn  MATLABFcn=0.5*u(3)+0.5*u(1)
  Logical Operator{,1..5} (6 alike) : Logic  AllPortsSameDT=off  OutDataTypeStr=boolean
  Logical Operator6 : Logic  Operator=OR  AllPortsSameDT=off  OutDataTypeStr=boolean
  Logical Operator7 : Logic  Operator=OR  AllPortsSameDT=off  OutDataTypeStr=boolean
  Logical Operator8 : Logic  Operator=OR  AllPortsSameDT=off  OutDataTypeStr=boolean
  Mux : Mux
  Relational Operator{,1..6} (7 alike) : RelationalOperator  Operator=<  OutDataTypeStr=boolean  RndMeth=Simplest
  Relational Operator{7..12} (6 alike) : RelationalOperator  OutDataTypeStr=boolean  RndMeth=Simplest
  VI : Outport
  wires:
  Mux/1 -> VI/1
  Data Type Conversion3/1 -> Mux/4
  Data Type Conversion2/1 -> Mux/3
  Data Type Conversion1/1 -> Mux/2
  Data Type Conversion/1 -> Mux/1
  Gain/1 -> Data Type Conversion/1
  Gain1/1 -> Data Type Conversion1/1
  Gain2/1 -> Data Type Conversion2/1
  Gain3/1 -> Data Type Conversion3/1
  Logical Operator3/1 -> Gain3/1
  Logical Operator8/1 -> Gain2/1
  Logical Operator7/1 -> Gain1/1
  Logical Operator6/1 -> Gain/1
  Logical Operator2/1 -> Logical Operator8/2
  Logical Operator4/1 -> Logical Operator8/1
  Logical Operator1/1 -> Logical Operator7/2
  Logical Operator5/1 -> Logical Operator7/1
  Logical Operator/1 -> Logical Operator6/2
  Relational Operator/1 -> Logical Operator6/1
  ramp/1 -> Relational Operator/1, Relational Operator1/1, Relational Operator2/1, Relational Operator3/1, Relational Operator4/1, Relational Operator5/1, Relational Operator6/1, Relational Operator7/1, Relational Operator8/1, Relational Operator9/1, Relational Operator10/1, Relational Operator11/1, Relational Operator12/1
  Relational Operator5/1 -> Logical Operator1/2
  Relational Operator8/1 -> Logical Operator1/1
  Relational Operator4/1 -> Logical Operator2/2
  Relational Operator9/1 -> Logical Operator2/1
  Relational Operator3/1 -> Logical Operator3/2
  Relational Operator10/1 -> Logical Operator3/1
  Relational Operator2/1 -> Logical Operator4/2
  Relational Operator11/1 -> Logical Operator4/1
  Relational Operator1/1 -> Logical Operator5/2
  Relational Operator12/1 -> Logical Operator5/1
  Relational Operator6/1 -> Logical Operator/2
  Relational Operator7/1 -> Logical Operator/1
  Interpreted MATLAB Function4/1 -> Relational Operator5/2, Relational Operator7/2
  Interpreted MATLAB Function5/1 -> Relational Operator6/2
  Interpreted MATLAB Function3/1 -> Relational Operator4/2, Relational Operator8/2
  Interpreted MATLAB Function2/1 -> Relational Operator3/2, Relational Operator9/2
  Interpreted MATLAB Function1/1 -> Relational Operator2/2, Relational Operator10/2
  Interpreted MATLAB Function6/1 -> Relational Operator1/2, Relational Operator11/2
  Interpreted MATLAB Function/1 -> Relational Operator/2, Relational Operator12/2
  Txy-07/1 -> Interpreted MATLAB Function/1, Interpreted MATLAB Function6/1, Interpreted MATLAB Function1/1, Interpreted MATLAB Function2/1, Interpreted MATLAB Function3/1, Interpreted MATLAB Function4/1, Interpreted MATLAB Function5/1
